simulink model "rocky_motor_disturb"  (R2021a)
settings: Solver=VariableStepAuto  StartTime=0.0  StopTime=2  RelTol=1e-3
model workspace (MAT data in the model file):
  m = 1000
values from neighbouring files (symbols this model uses):
  ci = -264    [rocky_constants.m]
  g = 9.8    [rocky_constants.m]
  ji = -516    [rocky_constants.m]
  jp = 33.67    [rocky_constants.m]
  ki = 8800    [rocky_constants.m]
  kmotor = .0025    (= 0.0025)    [rocky_constants.m]
  kp = 1000    [rocky_constants.m]
  l = 0.4822    [rocky_constants.m]
  tau = .103    (= 0.103)    [rocky_constants.m]
settings Model: Creator=clee1  LastModifiedBy=sdutta
settings SolverCC: AlgebraicLoopSolver=TrustRegion
settings DebuggingCC: SFMachineParentedDataDiag=warning

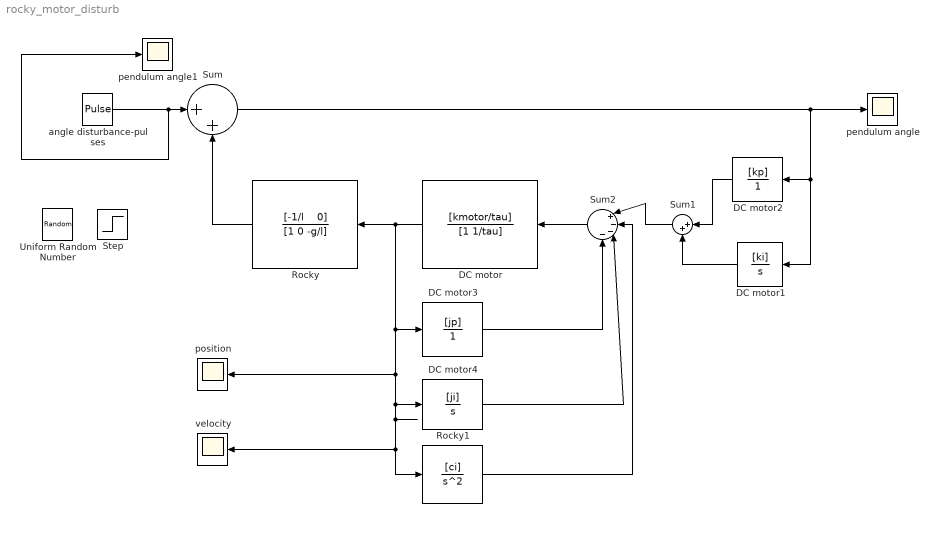
== system rocky_motor_disturb ==
  DC motor : TransferFcn  Numerator=[kmotor/tau]  Denominator=[1 1/tau]
  DC motor1 : TransferFcn  Numerator=[ki]  Denominator=[1 0]
  DC motor2 : TransferFcn  Numerator=[kp]  Denominator=[0 1]
  DC motor3 : TransferFcn  Numerator=[jp]  Denominator=[0 1]
  DC motor4 : TransferFcn  Numerator=[ji]  Denominator=[1 0]
  Rocky : TransferFcn  Numerator="[-1/l    0]"  Denominator=[1 0 -g/l]
  Rocky1 : TransferFcn  Numerator=[ci]  Denominator=[1 0 0]
  Step : Step  After=.1  SampleTime=0
  Sum : Sum  Inputs=|++
  Sum1 : Sum  Inputs=|++
  Sum2 : Sum  Inputs=|+---
  Uniform Random Number : UniformRandomNumber  SampleTime=20
  angle disturbance-pulses : DiscretePulseGenerator  PulseType=Time based  Amplitude=.1  Period=10  PulseWidth=.1  PhaseDelay=.5
  pendulum angle : Scope
  pendulum angle1 : Scope
  position : Scope
  "velocity " : Scope
  wires:
  Rocky/1 -> Sum/2
  Sum/1 -> DC motor1/1, DC motor2/1, pendulum angle/1
  angle disturbance-pulses/1 -> pendulum angle1/1, Sum/1
  DC motor/1 -> "velocity "/1, Rocky1/1, DC motor4/1, position/1, DC motor3/1, Rocky/1
  Sum2/1 -> DC motor/1
  DC motor2/1 -> Sum1/1
  DC motor1/1 -> Sum1/2
  Sum1/1 -> Sum2/1
  DC motor3/1 -> Sum2/4
  DC motor4/1 -> Sum2/3
  Rocky1/1 -> Sum2/2
